simulink model "fft"  (R2017a)
settings: Solver=VariableStepAuto  StartTime=0.0  StopTime=10.0  RelTol=1e-3
settings Model: Creator=guo  LastModifiedBy=guo

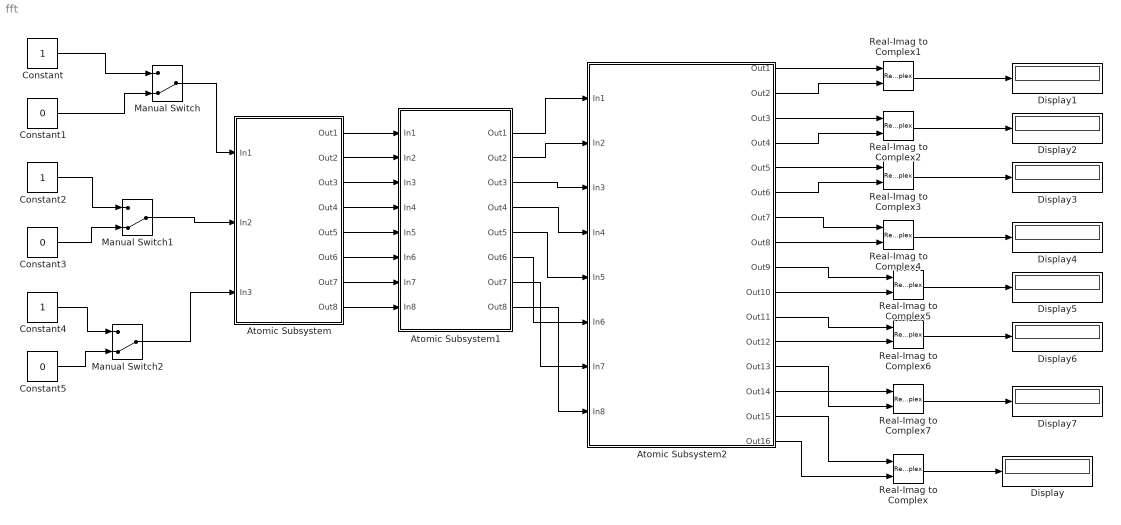
== system fft ==
  Atomic Subsystem : Subsystem  TreatAsAtomicUnit=on
  Atomic Subsystem1 : Subsystem  TreatAsAtomicUnit=on
  Atomic Subsystem2 : Subsystem  TreatAsAtomicUnit=on
  Constant : Constant
  Constant1 : Constant  Value=0
  Constant2 : Constant
  Constant3 : Constant  Value=0
  Constant4 : Constant
  Constant5 : Constant  Value=0
  Display{,1..7} (8 alike) : Display
  Manual Switch : ManualSwitch  CurrentSetting=0
  Manual Switch1 : ManualSwitch  CurrentSetting=0
  Manual Switch2 : ManualSwitch  CurrentSetting=0
  Real-Imag to Complex{,1..7} (8 alike) : RealImagToComplex
  wires:
  Constant/1 -> Manual Switch/1
  Constant1/1 -> Manual Switch/2
  Constant2/1 -> Manual Switch1/1
  Constant3/1 -> Manual Switch1/2
  Constant4/1 -> Manual Switch2/1
  Constant5/1 -> Manual Switch2/2
  Manual Switch/1 -> Atomic Subsystem/1(In1)
  Manual Switch1/1 -> Atomic Subsystem/2(In2)
  Manual Switch2/1 -> Atomic Subsystem/3(In3)
  Atomic Subsystem/1(Out1) -> Atomic Subsystem1/1(In1)
  Atomic Subsystem/2(Out2) -> Atomic Subsystem1/2(In2)
  Atomic Subsystem/3(Out3) -> Atomic Subsystem1/3(In3)
  Atomic Subsystem/4(Out4) -> Atomic Subsystem1/4(In4)
  Atomic Subsystem/5(Out5) -> Atomic Subsystem1/5(In5)
  Atomic Subsystem/6(Out6) -> Atomic Subsystem1/6(In6)
  Atomic Subsystem/7(Out7) -> Atomic Subsystem1/7(In7)
  Atomic Subsystem/8(Out8) -> Atomic Subsystem1/8(In8)
  Atomic Subsystem1/1(Out1) -> Atomic Subsystem2/1(In1)
  Atomic Subsystem1/2(Out2) -> Atomic Subsystem2/2(In2)
  Atomic Subsystem1/3(Out3) -> Atomic Subsystem2/3(In3)
  Atomic Subsystem1/4(Out4) -> Atomic Subsystem2/4(In4)
  Atomic Subsystem1/5(Out5) -> Atomic Subsystem2/5(In5)
  Atomic Subsystem1/6(Out6) -> Atomic Subsystem2/6(In6)
  Atomic Subsystem1/7(Out7) -> Atomic Subsystem2/7(In7)
  Atomic Subsystem1/8(Out8) -> Atomic Subsystem2/8(In8)
  Atomic Subsystem2/1(Out1) -> Real-Imag to Complex1/1
  Atomic Subsystem2/2(Out2) -> Real-Imag to Complex1/2
  Atomic Subsystem2/3(Out3) -> Real-Imag to Complex2/1
  Atomic Subsystem2/4(Out4) -> Real-Imag to Complex2/2
  Atomic Subsystem2/5(Out5) -> Real-Imag to Complex3/1
  Atomic Subsystem2/6(Out6) -> Real-Imag to Complex3/2
  Atomic Subsystem2/7(Out7) -> Real-Imag to Complex4/1
  Atomic Subsystem2/8(Out8) -> Real-Imag to Complex4/2
  Atomic Subsystem2/9(Out9) -> Real-Imag to Complex5/1
  Atomic Subsystem2/10(Out10) -> Real-Imag to Complex5/2
  Atomic Subsystem2/11(Out11) -> Real-Imag to Complex6/1
  Atomic Subsystem2/12(Out12) -> Real-Imag to Complex6/2
  Atomic Subsystem2/13(Out13) -> Real-Imag to Complex7/1
  Atomic Subsystem2/14(Out14) -> Real-Imag to Complex7/2
  Atomic Subsystem2/15(Out15) -> Real-Imag to Complex/1
  Atomic Subsystem2/16(Out16) -> Real-Imag to Complex/2
  Real-Imag to Complex1/1 -> Display1/1
  Real-Imag to Complex2/1 -> Display2/1
  Real-Imag to Complex3/1 -> Display3/1
  Real-Imag to Complex4/1 -> Display4/1
  Real-Imag to Complex5/1 -> Display5/1
  Real-Imag to Complex6/1 -> Display6/1
  Real-Imag to Complex7/1 -> Display7/1
  Real-Imag to Complex/1 -> Display/1

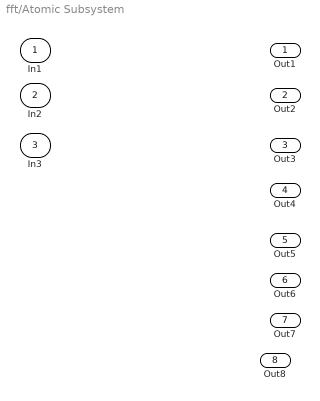
== system fft/Atomic Subsystem ==
  In1 : Inport
  In2 : Inport  Port=2
  In3 : Inport  Port=3
  Out1 : Outport
  Out2 : Outport  Port=2
  Out3 : Outport  Port=3
  Out4 : Outport  Port=4
  Out5 : Outport  Port=5
  Out6 : Outport  Port=6
  Out7 : Outport  Port=7
  Out8 : Outport  Port=8

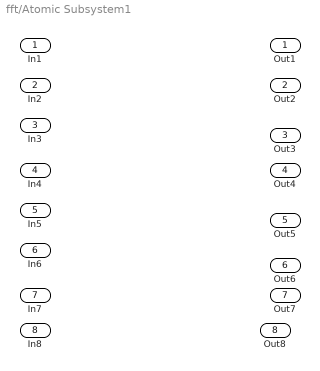
== system fft/Atomic Subsystem1 ==
  In1 : Inport
  In2 : Inport  Port=2
  In3 : Inport  Port=3
  In4 : Inport  Port=4
  In5 : Inport  Port=5
  In6 : Inport  Port=6
  In7 : Inport  Port=7
  In8 : Inport  Port=8
  Out1 : Outport
  Out2 : Outport  Port=2
  Out3 : Outport  Port=3
  Out4 : Outport  Port=4
  Out5 : Outport  Port=5
  Out6 : Outport  Port=6
  Out7 : Outport  Port=7
  Out8 : Outport  Port=8

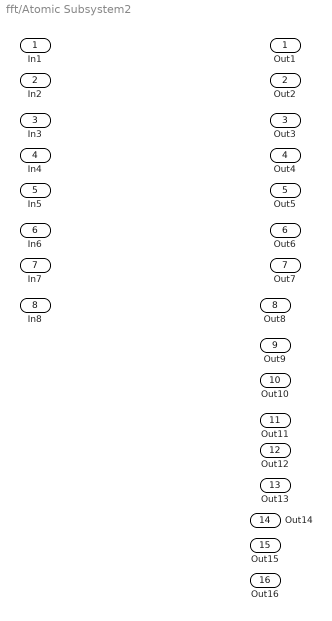
== system fft/Atomic Subsystem2 ==
  In1 : Inport
  In2 : Inport  Port=2
  In3 : Inport  Port=3
  In4 : Inport  Port=4
  In5 : Inport  Port=5
  In6 : Inport  Port=6
  In7 : Inport  Port=7
  In8 : Inport  Port=8
  Out1 : Outport
  Out2 : Outport  Port=2
  Out3 : Outport  Port=3
  Out4 : Outport  Port=4
  Out5 : Outport  Port=5
  Out6 : Outport  Port=6
  Out7 : Outport  Port=7
  Out8 : Outport  Port=8
  Out9 : Outport  Port=9
  Out10 : Outport  Port=10
  Out11 : Outport  Port=11
  Out12 : Outport  Port=12
  Out13 : Outport  Port=13
  Out14 : Outport  Port=14
  Out15 : Outport  Port=15
  Out16 : Outport  Port=16
